simulink model "LQI_obsv_hardware"  (R2024b)
settings: Solver=ode5  StartTime=0.0  StopTime=inf  FixedStep=dt  RelTol=1e-3
undefined symbols (not defined in the file): A, B, C, dt, Ki, Kx, L, National_Instruments, PCIe, r_pulley, x0, x_star
libraries: sldrtlib x4
settings Model: SimulationMode=external  Creator=johnc  LastModifiedBy=jcglenn
settings DataIOCC: MaxDataPoints=1000000
settings HardwareCC: ProdBitPerLong=64  ProdHWDeviceType=Intel->x86-64 (Linux 64)
settings RTWCC: Description=Simulink Desktop Real-Time (ERT)  SystemTargetFile=sldrtert.tlc  TemplateMakefile=sldrtert.tmf  RTWCompilerOptimization=on
settings CodeAppCC: MaxIdLength=95
settings SimulinkDesktopRealTimeERTCC: TargetFcnLib=ansi_tfl_table_tmw.mat  TargetLibSuffix=_sldrt.a  TargetPreCompLibLocation=C:\Program Files\MATLAB\R2024b\toolbox\sldrt\lib\win64  GenFloatMathFcnCalls=NOT IN USE  TargetLangStandard=C99 (ISO)  CodeReplacementLibrary=None  UtilityFuncGeneration=Auto  MultiwordTypeDef=System defined  MultiwordLength=2048  DynamicStringBufferSize=256  GenerateFullHeader=on  InferredTypesCompatibility=off  GenerateSampleERTMain=off  GenerateTestInterfaces=off  ModelReferenceCompliant=on  ParMdlRefBuildCompliant=on  CompOptLevelCompliant=on  ConcurrentExecutionCompliant=off  IncludeMdlTerminateFcn=on  CombineOutputUpdateFcns=off  CombineSignalStateStructs=off  GroupInternalDataByFunction=off  SuppressErrorStatus=off  IncludeFileDelimiter=Auto  ERTCustomFileBanners=off  SupportAbsoluteTime=on  LogVarNameModifier=rt_  MatFileLogging=off  CodeInterfacePackaging=Nonreusable function  PurelyIntegerCode=off  SupportNonFinite=on  SupportComplex=on  SupportContinuousTime=on  SupportNonInlinedSFcns=on  RemoveDisableFunc=off  RemoveResetFunc=off  SupportVariableSizeSignals=on  ParenthesesLevel=Nominal  CastingMode=Nominal  MATLABClassNameForMDSCustomization=Simulink.SoftwareTarget.TargetSpecificTriggerConfigurationBase  ModelStepFunctionPrototypeControlCompliant=off  CPPClassGenCompliant=off  AutosarCompliant=off  MDXCompliant=off  GRTInterface=off  GenerateAllocFcn=off  UseToolchainInfoCompliant=off  GenerateSharedConstants=on  CoderGroups=[]  AccessMethods=[]  LookupTableObjectStructAxisOrder=1,2,3,4,...  LUTObjectStructOrderExplicitValues=Size,Breakpoints,Table  LUTObjectStructOrderEvenSpacing=Size,Breakpoints,Table  ArrayLayout=Column-major  UnsupportedSFcnMsg=error  ERTHeaderFileRootName=$R$E  ERTSourceFileRootName=$R$E  ERTDataFileRootName=$R_data  InstructionSetFMA=off  OptimizeReductions=off  LogToMDFFile=off  GenerateASAP2=off  DSAsUniqueAccess=off  ExtMode=on  ExtModeTransport=0  ExtModeStaticAlloc=off  ExtModeAutomaticAllocSize=on  ExtModeMaxTrigDuration=10  ExtModeStaticAllocSize=1000000  ExtModeTesting=off  ExtModeMexFile=sldrtext  ExtModeIntrfLevel=Level1  InlinedParameterPlacement=Hierarchical  TargetOS=BareBoardExample  MultiInstanceErrorCode=Error  RootIOFormat=Individual arguments  RTWCAPISignals=off  RTWCAPIParams=off  RTWCAPIStates=off  RTWCAPIRootIO=off  ERTSrcFileBannerTemplate=ert_code_template.cgt  ERTHdrFileBannerTemplate=ert_code_template.cgt  ERTDataSrcFileTemplate=ert_code_template.cgt  ERTDataHdrFileTemplate=ert_code_template.cgt  ERTCustomFileTemplate=example_file_process.tlc  EnableDataOwnership=off  SignalDisplayLevel=10  ParamTuneLevel=10  GlobalDataDefinition=Auto  DataDefinitionFile=global.c  GlobalDataReference=Auto  ERTFilePackagingFormat=Modular  RateTransitionBlockCode=Inline  DataReferenceFile=global.h  PreserveExpressionOrder=off  PreserveIfCondition=off  ConvertIfToSwitch=off  PreserveExternInFcnDecls=on  PreserveStaticInFcnDecls=on  SuppressUnreachableDefaultCases=off  EnableSignedLeftShifts=on  EnableSignedRightShifts=on  ImplementImageWithCVMat=off  IndentStyle=K&R  IndentSize=2  NewlineStyle=Default  MaxLineWidth=80  EnableUserReplacementTypes=off  MaxIdInt64=MAX_int64_T  MinIdInt64=MIN_int64_T  MaxIdUint64=MAX_uint64_T  MaxIdInt32=MAX_int32_T  MinIdInt32=MIN_int32_T  MaxIdUint32=MAX_uint32_T  MaxIdInt16=MAX_int16_T  MinIdInt16=MIN_int16_T  MaxIdUint16=MAX_uint16_T  MaxIdInt8=MAX_int8_T  MinIdInt8=MIN_int8_T  MaxIdUint8=MAX_uint8_T  BooleanTrueId=true  BooleanFalseId=false  MemSecPackage=--- None ---  MemSecDataConstants=Default  MemSecDataIO=Default  MemSecDataInternal=Default  MemSecDataParameters=Default  MemSecFuncInitTerm=Default  MemSecFuncExecute=Default  MemSecFuncSharedUtil=Default  GroupConstants=Default  GroupRootInputs=Default  GroupRootOutputs=Default  GroupInternal=Default  GroupParameters=Default  GroupDataTransfer=Default  GroupSharedLocalDataStores=Default  GroupInstanceSpecificParameters=Default  GroupModelData=Default  ArrayContainerType=C-style array  DynamicArrayContainerType=std::vector  CCListing=off  RebuildAll=off

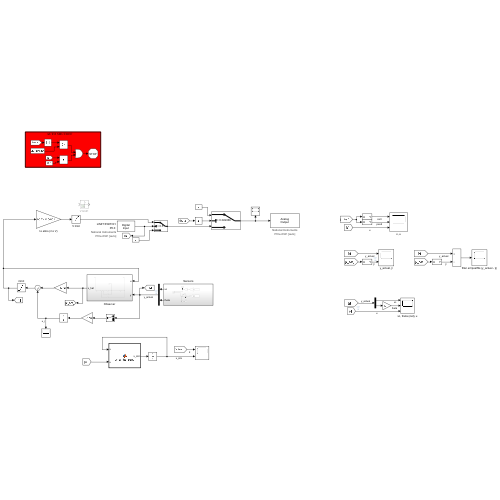
[thumbnail: Simulink's stored preview of the top-level diagram]
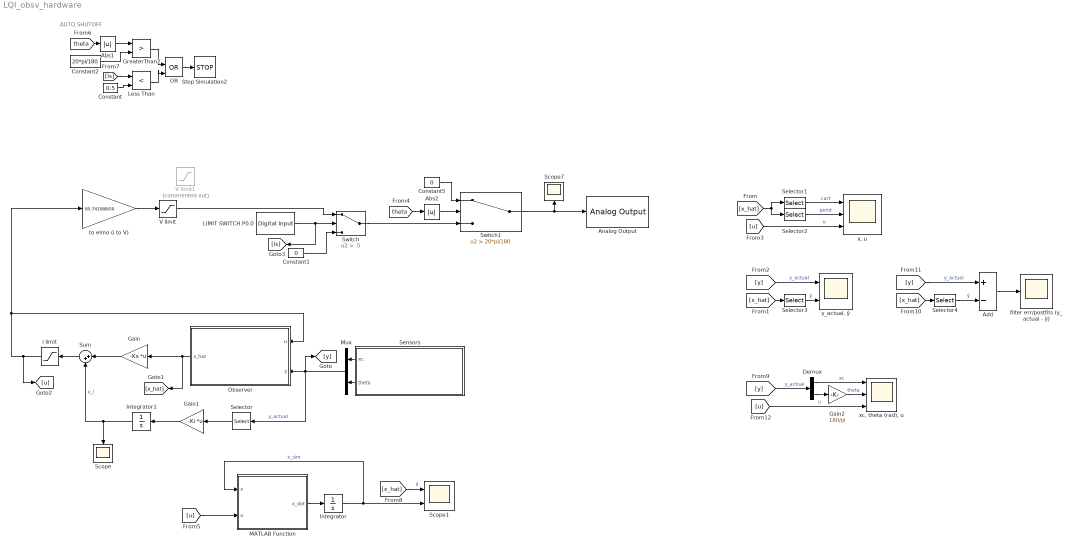
== system LQI_obsv_hardware ==
  note: AUTO SHUTOFF
  Abs1 : Abs  SaturateOnIntegerOverflow=off
  Abs2 : Abs  SaturateOnIntegerOverflow=off
  Add : Sum  Inputs=+-
  Analog Output : sldrtlib/Analog Output  SampleTime=dt  MaxMissedTicks=10  ShowMissedTicks=off  YieldWhenWaiting=off  DrvName=National_Instruments/PCIe-6321  DrvAddress=4294967295  DrvOptions=[0 0 0 2 2 3 0]  Channels=1  RangeMode=1  VoltRange=1  InitialValue=[0]  FinalValue=[0]
      settings: AttributesFormatString=National Instruments\nPCIe-6321 [auto]
  Constant : Constant  Value=0.5
  Constant1 : Constant  Value=0
  Constant2 : Constant  Value=20*pi/180
  Constant5 : Constant  Value=0
  Demux : Demux  Outputs=2
  Gain : Gain  Gain=-Kx  Multiplication=Matrix(K*u)
  Gain1 : Gain  Gain=-Ki  Multiplication=Matrix(K*u)
  Gain2 : Gain  Gain=180/pi
  GreaterThan2 : RelationalOperator  Operator=>  OutDataTypeStr=boolean  RndMeth=Simplest  InputSameDT=off
  Integrator : Integrator  InitialCondition=x0
  Integrator1 : Integrator
  LIMIT SWITCH P0.0 : sldrtlib/Digital Input  SampleTime=dt  MaxMissedTicks=10  ShowMissedTicks=off  YieldWhenWaiting=off  DrvName=National_Instruments/PCIe-6321  DrvAddress=4294967295  DrvOptions=[0 0 0 2 2 3 0]  Channels=1  BitMode=1  DataType=1
      settings: AttributesFormatString=National Instruments\nPCIe-6321 [auto]
  Less Than : RelationalOperator  Operator=<  OutDataTypeStr=boolean  RndMeth=Simplest  InputSameDT=off
  MATLAB Function : MATLAB Function  TreatAsAtomicUnit=on
  Mux : Mux  Inputs=2
  OR : Logic  Operator=OR  IconShape=distinctive  AllPortsSameDT=off  OutDataTypeStr=boolean
  Observer : Subsystem
  Scope : Scope
  Scope1 : Scope  NumInputPorts=2
  Scope7 : Scope
  Selector : Selector  InputPortWidth=2  IndexOptions=Index vector (dialog)  Indices=[1]  OutputSizes=1
  Selector1 : Selector  InputPortWidth=4  IndexOptions=Index vector (dialog)  Indices=[1 2]  OutputSizes=1
  Selector2 : Selector  InputPortWidth=4  IndexOptions=Index vector (dialog)  Indices=[3 4]  OutputSizes=1
  Selector3 : Selector  InputPortWidth=4  IndexOptions=Index vector (dialog)  Indices=[1 3]  OutputSizes=1
  Selector4 : Selector  InputPortWidth=4  IndexOptions=Index vector (dialog)  Indices=[1 3]  OutputSizes=1
  Sensors : Subsystem
  Stop Simulation2 : Stop
  Sum : Sum  Inputs=|++
  Switch : Switch  Criteria=u2 > Threshold  Threshold=.5  SaturateOnIntegerOverflow=off  InputSameDT=off
  Switch1 : Switch  Criteria=u2 > Threshold  Threshold=20*pi/180  SaturateOnIntegerOverflow=off  InputSameDT=off
  V limit : Saturate  UpperLimit=8.7455  LowerLimit=-8.7455
  V limit1 : Saturate  Commented=on  UpperLimit=9.75  LowerLimit=-9.75
  filter err/postfits (y_actual - ŷ) : Scope
  i limit : Saturate  UpperLimit=5.1  LowerLimit=-5.1
  to elmo (i to V) : Gain  Gain=85.741088/50
  "x, u" : Scope  NumInputPorts=3
  "xc, theta (rad), u" : Scope  NumInputPorts=3
  "y_actual, ŷ" : Scope  NumInputPorts=2
  wires:
  Observer/1(x_hat) -> Gain/1, [x_hat]
  [x_hat] -> Selector1/1, Selector2/1
  Selector1/1 -> "x, u"/1  "cart"
  Selector2/1 -> "x, u"/2  "pend"
  [y] -> "y_actual, ŷ"/1  "y_actual"
  [x_hat] -> Selector3/1
  [u] -> "x, u"/3  "u"
  Mux/1 -> Selector/1, Observer/2(y), [y]  "y_actual"
  Sensors/1(xc) -> Mux/1
  Sensors/2(theta) -> Mux/2
  Gain/1 -> Sum/1
  to elmo (i to V)/1 -> V limit/1
  [theta] -> Abs2/1
  Constant5/1 -> Switch1/1
  Abs2/1 -> Switch1/2
  Switch/1 -> Switch1/3
  LIMIT SWITCH P0.0/1 -> Switch/2, [ls]
  Constant1/1 -> Switch/3
  Switch1/1 -> Analog Output/1, Scope7/1
  V limit/1 -> Switch/1
  Constant2/1 -> GreaterThan2/2
  Abs1/1 -> GreaterThan2/1
  [theta] -> Abs1/1
  GreaterThan2/1 -> OR/1
  MATLAB Function/1(x_dot) -> Integrator/1
  Integrator/1 -> Scope1/2, MATLAB Function/1(x)  "x_sim"
  [u] -> MATLAB Function/2(u)
  Constant/1 -> Less Than/2
  Less Than/1 -> OR/2
  OR/1 -> Stop Simulation2/1
  [ls] -> Less Than/1
  [x_hat] -> Scope1/1  "x̂"
  Selector3/1 -> "y_actual, ŷ"/2  "ŷ"
  Sum/1 -> i limit/1
  Selector/1 -> Gain1/1
  Gain1/1 -> Integrator1/1
  i limit/1 -> [u], to elmo (i to V)/1, Observer/1(u)
  Integrator1/1 -> Scope/1, Sum/2  "u_i"
  [y] -> Demux/1  "y_actual"
  Demux/1 -> "xc, theta (rad), u"/1  "xc"
  Demux/2 -> Gain2/1
  Gain2/1 -> "xc, theta (rad), u"/2  "theta"
  Selector4/1 -> Add/2  "ŷ"
  [x_hat] -> Selector4/1
  [y] -> Add/1  "y_actual"
  Add/1 -> filter err/postfits (y_actual - ŷ)/1
  [u] -> "xc, theta (rad), u"/3  "u"

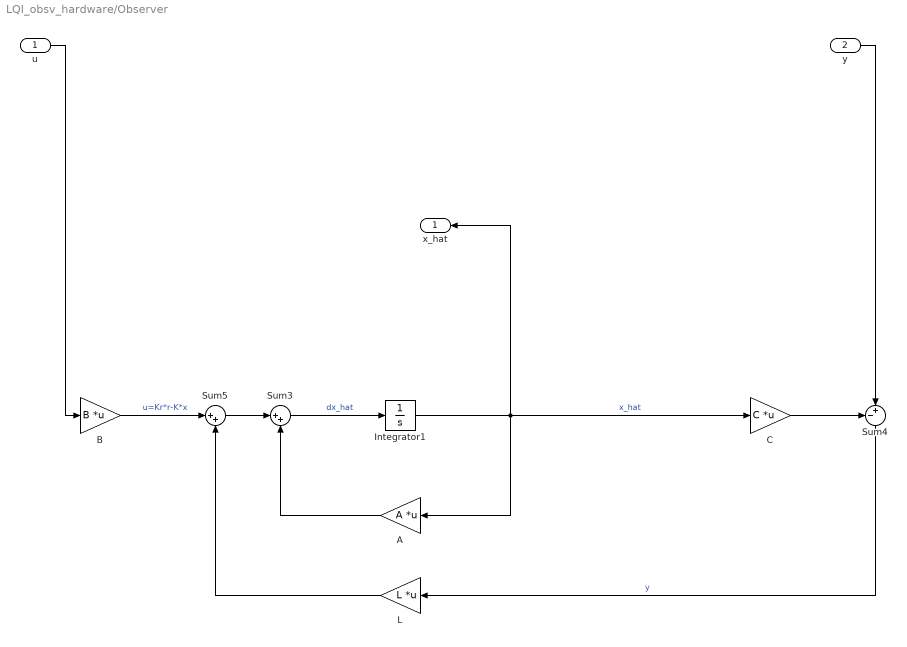
== system LQI_obsv_hardware/Observer ==
  u : Inport
  y : Inport  Port=2
  A : Gain  Gain=A  Multiplication=Matrix(K*u)
  B : Gain  Gain=B  Multiplication=Matrix(K*u)
  C : Gain  Gain=C  Multiplication=Matrix(K*u)
  Integrator1 : Integrator  InitialCondition=x0-x_star
  L : Gain  Gain=L  Multiplication=Matrix(K*u)
  Sum3 : Sum  Inputs=|++
  Sum4 : Sum  Inputs=-+|
  Sum5 : Sum  Inputs=|++
  x_hat : Outport
  wires:
  C/1 -> Sum4/1
  Integrator1/1 -> x_hat/1, C/1, A/1  "x_hat"
  Sum5/1 -> Sum3/1
  L/1 -> Sum5/2
  A/1 -> Sum3/2
  Sum4/1 -> L/1  "y"
  Sum3/1 -> Integrator1/1  "dx_hat"
  B/1 -> Sum5/1  "u=Kr*r-K*x"
  u/1 -> B/1
  y/1 -> Sum4/2

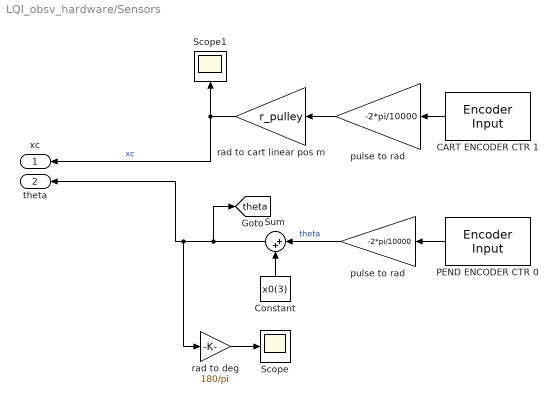
== system LQI_obsv_hardware/Sensors ==
  CART ENCODER CTR 1 : sldrtlib/Encoder Input  SampleTime=dt  MaxMissedTicks=10  ShowMissedTicks=off  YieldWhenWaiting=off  DrvName=National_Instruments/PCIe-6321  DrvAddress=4294967295  DrvOptions=[0 0 0 2 2 3 0]  Channels=2  QuadMode=3  IndexPulse=1  InputFilter=Inf  DataType=1
      settings: AttributesFormatString=National Instruments\nPCIe-6321 [auto]
  Constant : Constant  Value=x0(3)
  PEND ENCODER CTR 0 : sldrtlib/Encoder Input  SampleTime=dt  MaxMissedTicks=10  ShowMissedTicks=off  YieldWhenWaiting=off  DrvName=National_Instruments/PCIe-6321  DrvAddress=4294967295  DrvOptions=[0 0 0 2 2 3 0]  Channels=1  QuadMode=3  IndexPulse=1  InputFilter=Inf  DataType=1
      settings: AttributesFormatString=National Instruments\nPCIe-6321 [auto]
  Scope : Scope
  Scope1 : Scope
  Sum : Sum  Inputs=|++
  pulse to rad : Gain  Gain=-2*pi/10000
  "pulse to rad " : Gain  Gain=-2*pi/10000
  rad to cart linear pos m : Gain  Gain=r_pulley
  rad to deg : Gain  Gain=180/pi
  xc : Outport
  theta : Outport  Port=2
  tag scope: theta=global
  wires:
  rad to cart linear pos m/1 -> xc/1, Scope1/1  "xc"
  rad to deg/1 -> Scope/1
  PEND ENCODER CTR 0/1 -> pulse to rad/1
  "pulse to rad "/1 -> rad to cart linear pos m/1
  CART ENCODER CTR 1/1 -> "pulse to rad "/1
  Constant/1 -> Sum/2
  pulse to rad/1 -> Sum/1  "theta"
  Sum/1 -> [theta], rad to deg/1, theta/1

== matlab function LQI_obsv_hardware/MATLAB Function ==
  data: x input; x_dot output; u input; params parameter
function x_dot  = dynamics_pend(x, u, params)

g = params.g;
mc = params.mc;
mp = params.mp;
Jp = params.Jp;
bc = params.bc;
bp = params.bp;
Lp = params.Lp;
r_pulley = params.r_pulley;
Ke = params.Ke;

x1 = x(1);
x2 = x(2);
x3 = x(3);
x4 = x(4);

F_fric = 3*tanh(100*x2);
F_fric(abs(x2) < 2.5e-3) = 0;
F_fric = 0; % remove this dumbass

x1_dot = x2;
x2_dot = (Ke*u/r_pulley - bc*x2 - F_fric - mp*Lp*x4^2*sin(x3) + mp*Lp*cos(x3)*(-bp*x4 + mp*g*Lp*sin(x3))/(mp*Lp^2 + Jp))*1/(mc + mp - mp^2*Lp^2*cos(x3)^2/(mp*Lp^2 + Jp));
x3_dot = x4;
x4_dot = (-bp*x4 + mp*g*Lp*sin(x3) + mp*Lp*cos(x3)*(Ke*u/r_pulley - bc*x2 - mp*Lp*x4^2*sin(x3))/(mc + mp))*1/(mp*Lp^2 + Jp - mp^2*Lp^2*cos(x3)^2/(mc + mp));

x_dot = [x1_dot; x2_dot; x3_dot; x4_dot];
